simulink model "modular_airport_sim"  (R2021a)
settings: Solver=VariableStepAuto  StartTime=0.0  StopTime=1e6  RelTol=1e-3
undefined symbols (not defined in the file): m, n
settings Model: Creator=hagarusama  LastModifiedBy=hagarusama

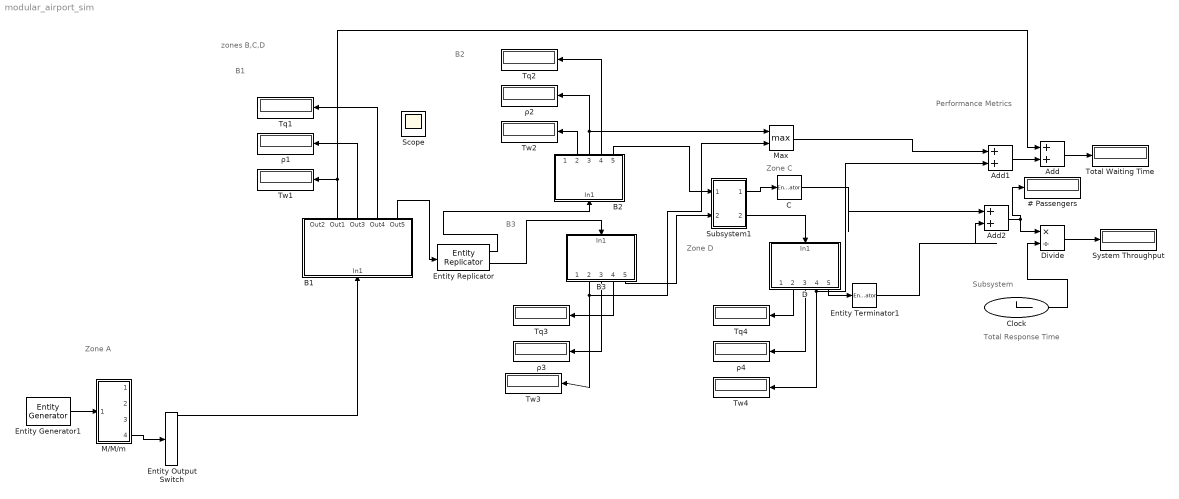
== system modular_airport_sim ==
  note: Zone A
  note: Zone C
  note: B3
  note: B2
  note: Zone D
  note: B1
  note: Performance Metrics
  note: Subsystem
  note: zones B,C,D
  note: Total Response Time
  # Passengers : Display
  Add : Sum
  Add1 : Sum
  Add2 : Sum
  B1 : Subsystem
  B2 : Subsystem
  B3 : Subsystem
  C : EntityTerminator  InputPortMessageModes=m  NumberEntitiesArrived=on
      settings: OutputPortMap=o0
  Clock : Clock
  D : Subsystem
  Divide : Product  Inputs=*/
  Entity Output Switch : EntityOutputSwitch  InputPortMessageModes=m  OutputPortMessageModes=m,m,m,m,m  NumberOutputPorts=5  SwitchingCriterion=Equiprobable  Seed=9647085  SwitchAttributeName=Attribute1
      settings: OutputPortMap=o0,o1,o2,o3,o4
  Entity Generator1 : EntityGenerator  OutputPortMessageModes=m  TimeSource=MATLAB action  IntergenerationTimeAction=|  GenerateAction=|  AttributeName=suspect  EntityType=Structured  EntityTypeName=Entity
      IntergenerationTimeAction=|
      | dt = rand(1,1);
      | persistent rngInit;
      | if isempty(rngInit)
      |     seed = 153503;
      |     rng(seed);
      |     rngInit = true;
      | end
      | 
      | % Pattern: Exponential distribution
      | mu = 1;
      | dt = -mu * log(1 - rand());
      GenerateAction=|
      | if 0.02 <= rand()
      |   entity.suspect = 1;
      | else
      |    entity.suspect = 2;
      | end
  Entity Replicator : EntityReplicator  InputPortMessageModes=m  OutputPortMessageModes=m,m
  Entity Terminator1 : EntityTerminator  InputPortMessageModes=m  NumberEntitiesArrived=on
      settings: OutputPortMap=o0
  M/M/m : Subsystem
  Max : MinMax  Function=max  Inputs=2
  Subsystem1 : Subsystem
  System Throughput : Display
  Total Waiting Time : Display
  Tq{1..4} (4 alike) : Display
  Tw{1..4} (4 alike) : Display
  ρ{1..4} (4 alike) : Display
  Scope : Scope
  wires:
  Subsystem1/1(Out1) -> C/1
  Entity Generator1/1 -> M/M/m/1(In1)
  M/M/m/4(Out4) -> Entity Output Switch/1
  Entity Output Switch/1 -> B1/1(In1)
  Entity Replicator/1 -> B2/1(In1)
  Entity Replicator/2 -> B3/1(In1)
  B2/5(Out5) -> Subsystem1/1(In1)
  B3/5(Out5) -> Subsystem1/2(In2)
  Subsystem1/2(Out2) -> D/1(In1)
  B1/3(Out3) -> ρ1/1
  B1/4(Out4) -> Tq1/1
  B2/2(Out1) -> Tw2/1
  B2/3(Out3) -> ρ2/1, Max/1
  B2/4(Out4) -> Tq2/1
  B3/2(Out1) -> Tw3/1, Max/2
  B3/3(Out3) -> ρ3/1
  B3/4(Out4) -> Tq3/1
  D/5(Out5) -> Entity Terminator1/1
  D/2(Out1) -> Tq4/1
  D/3(Out3) -> ρ4/1
  D/4(Out4) -> Tw4/1, Add1/2
  B1/2(Out1) -> Add/1, Tw1/1
  Add1/1 -> Add/2
  Max/1 -> Add1/1
  Add/1 -> Total Waiting Time/1
  Entity Terminator1/1 -> Add2/2
  C/1 -> Add2/1
  Add2/1 -> # Passengers/1, Divide/1
  Clock/1 -> Divide/2
  Divide/1 -> System Throughput/1
  B1/5(Out5) -> Entity Replicator/1

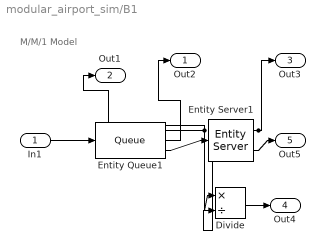
== system modular_airport_sim/B1 ==
  note: M/M/1 Model
  In1 : Inport
  Divide : Product  Inputs=*/
  Entity Queue1 : Queue  InputPortMessageModes=m  OutputPortMessageModes=n,n,m  Capacity=inf  AverageWait=on  AverageQueueLength=on
      settings: OutputPortMap=o2,o3,o5
  Entity Server1 : EntityServer  InputPortMessageModes=m  OutputPortMessageModes=n,m  Capacity=1  ServiceTimeSource=MATLAB action  ServiceTimeAction=|  Utilization=on
      | dt = rand(1,1);
      | persistent rngInit;
      | if isempty(rngInit)
      |     seed = 2273520;
      |     rng(seed);
      |     rngInit = true;
      | end
      | 
      | % Pattern: Exponential distribution
      | mu = 10;
      | dt = -mu * log(1 - rand());
      settings: OutputPortMap=o5,o9
  Out2 : Outport
  Out1 : Outport  Port=2
  Out3 : Outport  Port=3
  Out4 : Outport  Port=4
  Out5 : Outport  Port=5
  wires:
  In1/1 -> Entity Queue1/1
  Entity Queue1/2 -> Out2/1
  Entity Server1/1 -> Divide/2, Out3/1
  Entity Queue1/1 -> Divide/1, Out1/1
  Entity Queue1/3 -> Entity Server1/1
  Entity Server1/2 -> Out5/1
  Divide/1 -> Out4/1

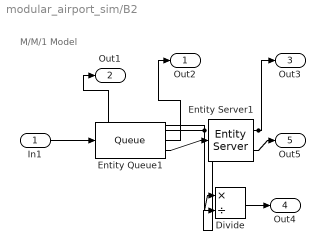
== system modular_airport_sim/B2 ==
  note: M/M/1 Model
  In1 : Inport
  Divide : Product  Inputs=*/
  Entity Queue1 : Queue  InputPortMessageModes=m  OutputPortMessageModes=n,n,m  Capacity=inf  AverageWait=on  AverageQueueLength=on
      settings: OutputPortMap=o2,o3,o5
  Entity Server1 : EntityServer  InputPortMessageModes=m  OutputPortMessageModes=n,m  Capacity=1  ServiceTimeSource=MATLAB action  ServiceTimeAction=|  Utilization=on
      | dt = rand(1,1);
      | persistent rngInit;
      | if isempty(rngInit)
      |     seed = 7612432;
      |     rng(seed);
      |     rngInit = true;
      | end
      | 
      | % Pattern: Exponential distribution
      | mu = 3;
      | dt = -mu * log(1 - rand());
      settings: OutputPortMap=o5,o9
  Out2 : Outport
  Out1 : Outport  Port=2
  Out3 : Outport  Port=3
  Out4 : Outport  Port=4
  Out5 : Outport  Port=5
  wires:
  Divide/1 -> Out4/1
  Entity Server1/2 -> Out5/1
  Entity Queue1/3 -> Entity Server1/1
  Entity Queue1/1 -> Out1/1, Divide/1
  Entity Server1/1 -> Out3/1, Divide/2
  Entity Queue1/2 -> Out2/1
  In1/1 -> Entity Queue1/1

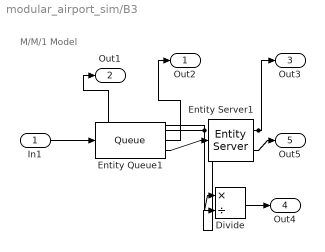
== system modular_airport_sim/B3 ==
  note: M/M/1 Model
  In1 : Inport
  Divide : Product  Inputs=*/
  Entity Queue1 : Queue  InputPortMessageModes=m  OutputPortMessageModes=n,n,m  Capacity=inf  AverageWait=on  AverageQueueLength=on
      settings: OutputPortMap=o2,o3,o5
  Entity Server1 : EntityServer  InputPortMessageModes=m  OutputPortMessageModes=n,m  Capacity=1  ServiceTimeSource=MATLAB action  ServiceTimeAction=|  Utilization=on
      | dt = rand(1,1);
      | persistent rngInit;
      | if isempty(rngInit)
      |     seed = 6069205;
      |     rng(seed);
      |     rngInit = true;
      | end
      | 
      | % Pattern: Exponential distribution
      | mu = 3;
      | dt = -mu * log(1 - rand());
      settings: OutputPortMap=o5,o9
  Out2 : Outport
  Out1 : Outport  Port=2
  Out3 : Outport  Port=3
  Out4 : Outport  Port=4
  Out5 : Outport  Port=5
  wires:
  In1/1 -> Entity Queue1/1
  Entity Queue1/2 -> Out2/1
  Entity Server1/1 -> Divide/2, Out3/1
  Entity Queue1/1 -> Divide/1, Out1/1
  Entity Queue1/3 -> Entity Server1/1
  Entity Server1/2 -> Out5/1
  Divide/1 -> Out4/1

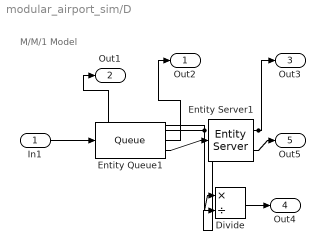
== system modular_airport_sim/D ==
  note: M/M/1 Model
  In1 : Inport
  Divide : Product  Inputs=*/
  Entity Queue1 : Queue  InputPortMessageModes=m  OutputPortMessageModes=n,n,m  Capacity=inf  AverageWait=on  AverageQueueLength=on
      settings: OutputPortMap=o2,o3,o5
  Entity Server1 : EntityServer  InputPortMessageModes=m  OutputPortMessageModes=n,m  Capacity=1  ServiceTimeSource=MATLAB action  ServiceTimeAction=|  Utilization=on
      | dt = rand(1,1);
      | persistent rngInit;
      | if isempty(rngInit)
      |     seed = 6069205;
      |     rng(seed);
      |     rngInit = true;
      | end
      | 
      | % Pattern: Exponential distribution
      | mu = 60;
      | dt = -mu * log(1 - rand());
      settings: OutputPortMap=o5,o9
  Out2 : Outport
  Out1 : Outport  Port=2
  Out3 : Outport  Port=3
  Out4 : Outport  Port=4
  Out5 : Outport  Port=5
  wires:
  Divide/1 -> Out4/1
  Entity Server1/2 -> Out5/1
  Entity Queue1/3 -> Entity Server1/1
  Entity Queue1/1 -> Out1/1, Divide/1
  Entity Server1/1 -> Out3/1, Divide/2
  Entity Queue1/2 -> Out2/1
  In1/1 -> Entity Queue1/1

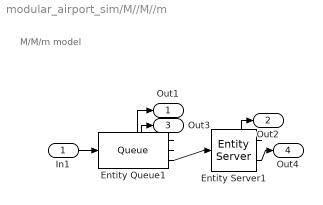
== system modular_airport_sim/M//M//m ==
  note: M/M/m model
  In1 : Inport
  Entity Queue1 : Queue  InputPortMessageModes=m  OutputPortMessageModes=n,n,m  Capacity=inf  AverageWait=on  AverageQueueLength=on
      settings: OutputPortMap=o2,o3,o5
  Entity Server1 : EntityServer  InputPortMessageModes=m  OutputPortMessageModes=n,m  ServiceTimeSource=MATLAB action  ServiceTimeAction=|  Utilization=on
      | dt = rand(1,1);
      | persistent rngInit;
      | if isempty(rngInit)
      |     seed = 8084213;
      |     rng(seed);
      |     rngInit = true;
      | end
      | 
      | % Pattern: Exponential distribution
      | mu = 1;
      | dt = -mu * log(1 - rand());
      settings: OutputPortMap=o5,o9
  Out1 : Outport
  Out2 : Outport  Port=2
  Out3 : Outport  Port=3
  Out4 : Outport  Port=4
  wires:
  Entity Queue1/3 -> Entity Server1/1
  Entity Queue1/1 -> Out3/1
  In1/1 -> Entity Queue1/1
  Entity Queue1/2 -> Out1/1
  Entity Server1/2 -> Out4/1
  Entity Server1/1 -> Out2/1

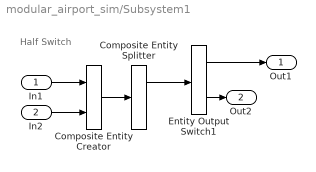
== system modular_airport_sim/Subsystem1 ==
  note: Half Switch
  In1 : Inport
  In2 : Inport  Port=2
  Composite Entity Creator : CompositeEntityCreator  InputPortMessageModes=m,m  OutputPortMessageModes=m  EntityTypeName=Combined
      settings: InputPortMap=u0,u1
  Composite Entity Splitter : CompositeEntitySplitter  InputPortMessageModes=m  OutputPortMessageModes=m,m
      settings: OutputPortMap=o0,o1
  Entity Output Switch1 : EntityOutputSwitch  InputPortMessageModes=m  OutputPortMessageModes=m,m  SwitchingCriterion=From attribute  Seed=9631392  SwitchAttributeName=entity.suspect
  Out1 : Outport
  Out2 : Outport  Port=2
  wires:
  Composite Entity Creator/1 -> Composite Entity Splitter/1
  Entity Output Switch1/2 -> Out2/1
  Composite Entity Splitter/1 -> Entity Output Switch1/1
  In2/1 -> Composite Entity Creator/2
  Entity Output Switch1/1 -> Out1/1
  In1/1 -> Composite Entity Creator/1
